simulink model "Ex0_2"  (R2019a)
settings: Solver=VariableStepAuto  StartTime=0.0  StopTime=20.0  RelTol=1e-3
values from neighbouring files (symbols this model uses):
  K = 1    [value0.m]
  T1 = 1    [value0.m]
  T2 = 2    [value0.m]
  T3 = 3    [value0.m]
settings Model: Creator=Takumi SHIOTA  LastModifiedBy=Takumi SHIOTA

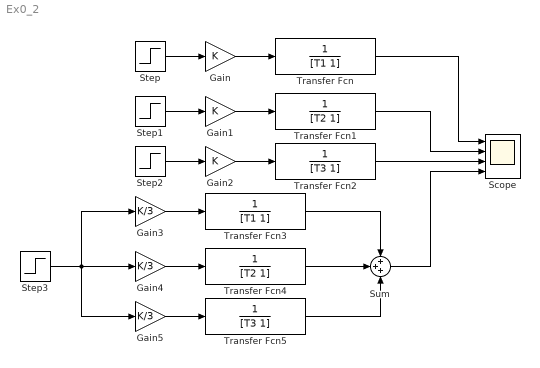
== system Ex0_2 ==
  Gain : Gain  Gain=K
  Gain1 : Gain  Gain=K
  Gain2 : Gain  Gain=K
  Gain3 : Gain  Gain=K/3
  Gain4 : Gain  Gain=K/3
  Gain5 : Gain  Gain=K/3
  Scope : Scope  NumInputPorts=4
  Step{,1..3} (4 alike) : Step  SampleTime=0
  Sum : Sum  Inputs=+++
  Transfer Fcn : TransferFcn  Denominator=[T1 1]
  Transfer Fcn1 : TransferFcn  Denominator=[T2 1]
  Transfer Fcn2 : TransferFcn  Denominator=[T3 1]
  Transfer Fcn3 : TransferFcn  Denominator=[T1 1]
  Transfer Fcn4 : TransferFcn  Denominator=[T2 1]
  Transfer Fcn5 : TransferFcn  Denominator=[T3 1]
  wires:
  Transfer Fcn2/1 -> Scope/3
  Transfer Fcn/1 -> Scope/1
  Step2/1 -> Gain2/1
  Gain/1 -> Transfer Fcn/1
  Gain1/1 -> Transfer Fcn1/1
  Step1/1 -> Gain1/1
  Step/1 -> Gain/1
  Gain2/1 -> Transfer Fcn2/1
  Transfer Fcn1/1 -> Scope/2
  Gain3/1 -> Transfer Fcn3/1
  Gain4/1 -> Transfer Fcn4/1
  Step3/1 -> Gain5/1, Gain3/1, Gain4/1
  Gain5/1 -> Transfer Fcn5/1
  Transfer Fcn3/1 -> Sum/1
  Transfer Fcn5/1 -> Sum/3
  Transfer Fcn4/1 -> Sum/2
  Sum/1 -> Scope/4
